simulink model "slm3"  (R2018a)
settings: Solver=VariableStepAuto  StartTime=0.0  StopTime=10.0  RelTol=1e-3
values from neighbouring files (symbols this model uses):
  B = 1    [setup.m]
  k = [.1,1,5]    [setup.m]
  X = 1    [setup.m]
settings Model: Creator=Pranav Maddula  LastModifiedBy=Pranav Maddula

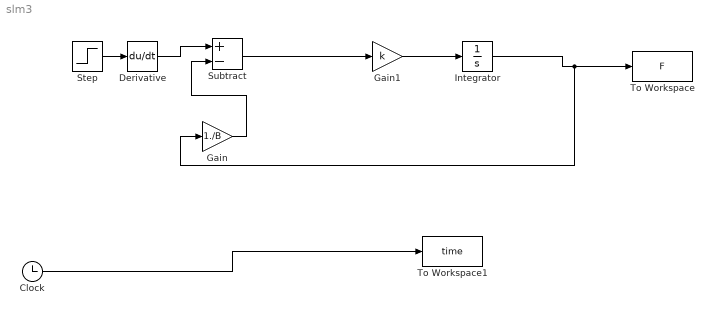
== system slm3 ==
  Clock : Clock
  Derivative : Derivative
  Gain : Gain  Gain=1./B
  Gain1 : Gain  Gain=k
  Integrator : Integrator
  Step : Step  After=X  SampleTime=0
  Subtract : Sum  Inputs=+-
  To Workspace : ToWorkspace  VariableName=F  SampleTime=-1
  To Workspace1 : ToWorkspace  VariableName=time  SampleTime=-1
  wires:
  Step/1 -> Derivative/1
  Derivative/1 -> Subtract/1
  Gain/1 -> Subtract/2
  Integrator/1 -> Gain/1, To Workspace/1
  Gain1/1 -> Integrator/1
  Subtract/1 -> Gain1/1
  Clock/1 -> To Workspace1/1
